simulink model "bh_solenoid_simulink_step_04"  (R2018a)
settings: Solver=ode45  StartTime=0.0  StopTime=3  FixedStep=1e-4  MaxStep=1e-4  RelTol=1e-5
undefined symbols (not defined in the file): Coeffs, Elec, Mech, sigbuilder_block, solen
settings Model: Creator=bhorton  LastModifiedBy=bhorton

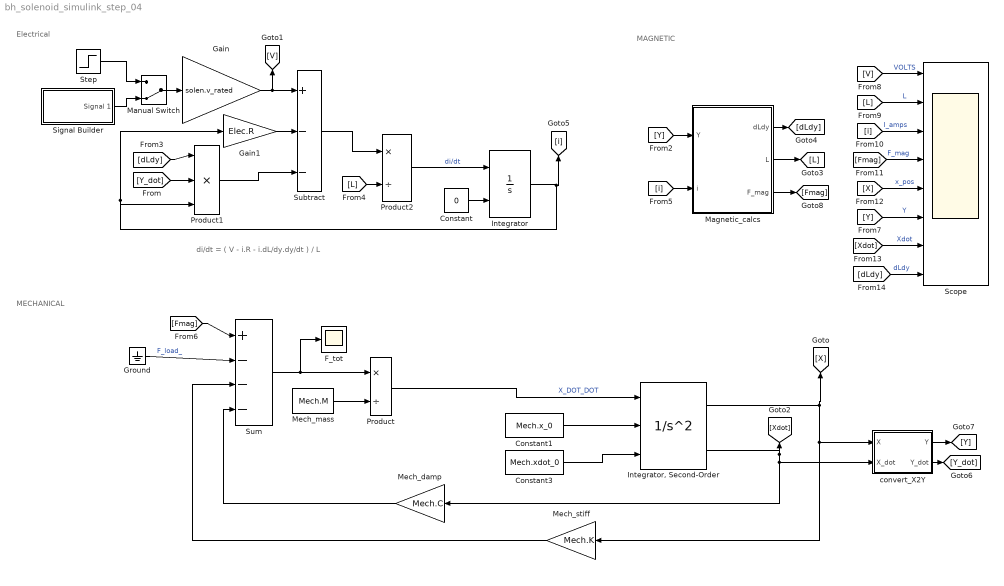
== system bh_solenoid_simulink_step_04 ==
  note: di/dt = ( V - i.R - i.dL/dy.dy/dt ) / L
  note: MAGNETIC
  note: Electrical
  note: MECHANICAL
  Constant : Constant  Value=0
  Constant1 : Constant  Value=Mech.x_0
  Constant3 : Constant  Value=Mech.xdot_0
  F_tot : Scope
  Gain : Gain  Gain=solen.v_rated
  Gain1 : Gain  Gain=Elec.R
  Ground : Ground
  Integrator : Integrator  InitialConditionSource=external
  "Integrator, Second-Order" : SecondOrderIntegrator  ICSourceX=external  LimitX=on  UpperLimitX=Mech.x_max  LowerLimitX=Mech.x_min  ICSourceDXDT=external
  Magnetic_calcs : Subsystem
  Manual Switch : ManualSwitch  CurrentSetting=0
  Mech_damp : Gain  Gain=Mech.C
  Mech_mass : Constant  Value=Mech.M
  Mech_stiff : Gain  Gain=Mech.K
  Product : Product  Inputs=*/
  Product1 : Product  Inputs=3
  Product2 : Product  Inputs=*/
  Scope : Scope  NumInputPorts=8
  Signal Builder : Subsystem  Tag=STV Subsys  LoadFcn=sigbuilder_block('load');  StartFcn=sigbuilder_block('start');  StopFcn=sigbuilder_block('stop');  ClipboardFcn=sigbuilder_block('clipboard');  mask(Sigbuilder block){tuvar=[0:10]}
      mask help: Simulink:masks:SigbuilderBlock_MD
      mask init:
      | if ~strcmp(get_param(bdroot(gcbh),'SimulationStatus'),'stopped') tuvar = sigbuilder_block('maskInit'); end
      settings: CopyFcn=sigbuilder_block('copy');  DeleteFcn=sigbuilder_block('delete');  ModelCloseFcn=sigbuilder_block('modelClose');  PreSaveFcn=sigbuilder_block('preSave');  PauseFcn=sigbuilder_block('pause');  ContinueFcn=sigbuilder_block('continue');  NameChangeFcn=sigbuilder_block('namechange');  OpenFcn=sigbuilder_block('open',[437.6 199.2 550.4 400 ]);  CloseFcn=sigbuilder_block('close');
      mask Display: plot(0, 0, 100, 100,[2, 2, 32, 32, 2], [68, 8, 8, 68, 68],[32, 2], [38, 38], [32, 19, 2],[53, 60, 44], [32, 17, 17, 2],[16, 16, 31, 31]);txt = getActiveGroup(gcbh);text(2, 100, txt,'verticalAlignment', 'top');
  Step : Step  Time=0.1  SampleTime=0
  Subtract : Sum  Inputs=+--
  Sum : Sum  Inputs=+|-|-|-
  convert_X2Y : Subsystem
  wires:
  Sum/1 -> F_tot/1, Product/1
  Mech_mass/1 -> Product/2
  Product/1 -> "Integrator, Second-Order"/1  "X_DOT_DOT"
  Mech_damp/1 -> Sum/4
  Mech_stiff/1 -> Sum/3
  Ground/1 -> Sum/2  "F_load_"
  [V] -> Scope/1  "VOLTS"
  [L] -> Scope/2  "L"
  [i] -> Scope/3  "I_amps"
  [Fmag] -> Scope/4  "F_mag"
  [X] -> Scope/5  "x_pos"
  Constant3/1 -> "Integrator, Second-Order"/3
  Constant1/1 -> "Integrator, Second-Order"/2
  "Integrator, Second-Order"/1 -> [X], convert_X2Y/1(X), Mech_stiff/1
  "Integrator, Second-Order"/2 -> Mech_damp/1, convert_X2Y/2(X_dot), [Xdot]
  convert_X2Y/1(Y) -> [Y]
  convert_X2Y/2(Y_dot) -> [Y_dot]
  Magnetic_calcs/3(F_mag) -> [Fmag]
  Magnetic_calcs/2(L) -> [L]
  Magnetic_calcs/1(dLdy) -> [dLdy]
  [Y] -> Magnetic_calcs/1(Y)
  [i] -> Magnetic_calcs/2(i)
  [Fmag] -> Sum/1
  [Y] -> Scope/6  "Y"
  [Xdot] -> Scope/7  "Xdot"
  [dLdy] -> Scope/8  "dLdy"
  Signal Builder/1(Signal 1) -> Manual Switch/2
  Step/1 -> Manual Switch/1
  Gain/1 -> Subtract/1, [V]
  Manual Switch/1 -> Gain/1
  Constant/1 -> Integrator/2
  Product2/1 -> Integrator/1  "di/dt"
  Subtract/1 -> Product2/1
  [L] -> Product2/2
  Integrator/1 -> [i], Product1/3, Gain1/1
  [dLdy] -> Product1/1
  [Y_dot] -> Product1/2
  Gain1/1 -> Subtract/2
  Product1/1 -> Subtract/3

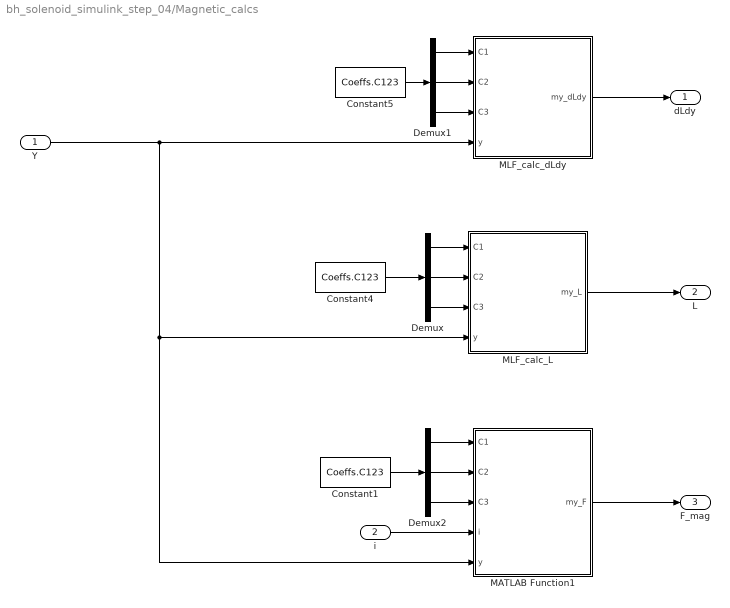
== system bh_solenoid_simulink_step_04/Magnetic_calcs ==
  Y : Inport
  i : Inport  Port=2
  Constant1 : Constant  Value=Coeffs.C123
  Constant4 : Constant  Value=Coeffs.C123
  Constant5 : Constant  Value=Coeffs.C123
  Demux : Demux  Outputs=3
  Demux1 : Demux  Outputs=3
  Demux2 : Demux  Outputs=3
  MATLAB Function1 : MATLAB Function  TreatAsAtomicUnit=on
  MLF_calc_L : MATLAB Function  TreatAsAtomicUnit=on
  MLF_calc_dLdy : MATLAB Function  TreatAsAtomicUnit=on
  dLdy : Outport
  L : Outport  Port=2
  F_mag : Outport  Port=3
  wires:
  Demux/2 -> MLF_calc_L/2(C2)
  Demux1/2 -> MLF_calc_dLdy/2(C2)
  Demux/3 -> MLF_calc_L/3(C3)
  Constant4/1 -> Demux/1
  Demux/1 -> MLF_calc_L/1(C1)
  Demux1/3 -> MLF_calc_dLdy/3(C3)
  Demux1/1 -> MLF_calc_dLdy/1(C1)
  Constant5/1 -> Demux1/1
  Y/1 -> MATLAB Function1/5(y), MLF_calc_L/4(y), MLF_calc_dLdy/4(y)
  MATLAB Function1/1(my_F) -> F_mag/1
  Demux2/1 -> MATLAB Function1/1(C1)
  Constant1/1 -> Demux2/1
  Demux2/3 -> MATLAB Function1/3(C3)
  Demux2/2 -> MATLAB Function1/2(C2)
  i/1 -> MATLAB Function1/4(i)
  MLF_calc_dLdy/1(my_dLdy) -> dLdy/1
  MLF_calc_L/1(my_L) -> L/1

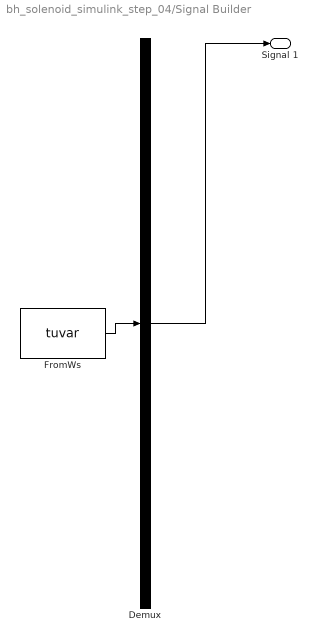
== system bh_solenoid_simulink_step_04/Signal Builder ==
  Demux : Demux  Tag=STV Demux  Outputs=1
  FromWs : FromWorkspace  Tag=STV FromWs  VariableName=tuvar  SampleTime=0
      SigBuilderData=|
      | common.afterFinalStr = 'Extrapolate'
      | common.sampleTime = 0
      | dataSet.timeRange = [0 2]
      | dataSet.name = 'Group 1'
      | sbobj.Groups.Name = 'Group 1'
      | sbobj.Groups.Signals.Name = 'Signal 1'
      | sbobj.Groups.Signals.XData = [0 0.1 0.1 1.5 1.5 2]
      | sbobj.Groups.Signals.YData = [0 0 1 1 0 0]
      | sbobj.Groups.TimeRange = [0 2]
  Signal 1 : Outport  Tag=STV Outport
  wires:
  Demux/1 -> Signal 1/1
  FromWs/1 -> Demux/1

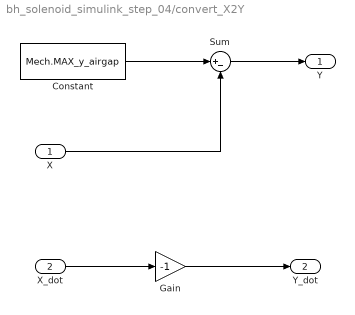
== system bh_solenoid_simulink_step_04/convert_X2Y ==
  X : Inport
  X_dot : Inport  Port=2
  Constant : Constant  Value=Mech.MAX_y_airgap
  Gain : Gain  Gain=-1
  Sum : Sum  Inputs=|+-
  Y : Outport
  Y_dot : Outport  Port=2
  wires:
  Constant/1 -> Sum/1
  X/1 -> Sum/2
  Sum/1 -> Y/1
  X_dot/1 -> Gain/1
  Gain/1 -> Y_dot/1

== matlab function bh_solenoid_simulink_step_04/Magnetic_calcs/MLF_calc_L ==
  data: C1 input; my_L output; C2 input; C3 input; y input
function my_L = calc_L(C1,C2,C3, y)

my_L = bh_func_calc_my_L(C1,C2,C3, y);

== matlab function bh_solenoid_simulink_step_04/Magnetic_calcs/MLF_calc_dLdy ==
  data: C1 input; my_dLdy output; C2 input; C3 input; y input
function my_dLdy = calc_dLdy(C1,C2,C3, y)

my_dLdy = bh_func_calc_my_dLdy(C1,C2,C3, y);

== matlab function bh_solenoid_simulink_step_04/Magnetic_calcs/MATLAB Function1 ==
  data: C1 input; my_F output; C2 input; C3 input; i input; y input
function my_F = calc_F(C1,C2,C3, i, y)

my_F = bh_func_calc_my_F(C1,C2,C3, i, y);
